simulink library "inp"  (R2021b)
settings: Solver=VariableStepAuto  StartTime=0.0  StopTime=10.0  RelTol=1e-3
undefined symbols (not defined in the file): C_TASK_5MS_S, FALSE, KINP_AcoreReadyToSlp_flg_ovrdflg, KINP_AcoreReadyToSlp_flg_ovrdval, KINP_AllowMovThd_OTA_enum_ovrdflg, KINP_AllowMovThd_OTA_enum_ovrdval, KINP_APSAngleTarget_Deg_ovrdflg, KINP_APSAngleTarget_Deg_ovrdval, KINP_APSDecReq_mps2_ovrdflg, KINP_APSDecReq_mps2_ovrdval, KINP_APSDecReqA_flg_ovrdflg, KINP_APSDecReqA_flg_ovrdval, KINP_APSDFLL_cm_ovrdflg, KINP_APSDFLL_cm_ovrdval, KINP_APSDFLR_cm_ovrdflg, KINP_APSDFLR_cm_ovrdval, KINP_APSDRLL_cm_ovrdflg, KINP_APSDRLL_cm_ovrdval, KINP_APSDRLR_cm_ovrdflg, KINP_APSDRLR_cm_ovrdval, KINP_APSExitCondition_enum_ovrdflg, KINP_APSExitCondition_enum_ovrdval, KINP_APSHWVer_enum_ovrdflg, KINP_APSHWVer_enum_ovrdval, KINP_APSProgressPCT_pct_ovrdflg, KINP_APSProgressPCT_pct_ovrdval, KINP_APSPwrReq_enum_ovrdflg, KINP_APSPwrReq_enum_ovrdval, KINP_APSReq_enum_ovrdflg, KINP_APSReq_enum_ovrdval, KINP_APSRQDisplay_enum_ovrdflg, KINP_APSRQDisplay_enum_ovrdval, KINP_APSRqEPASCtrl_flg_ovrdflg, KINP_APSRqEPASCtrl_flg_ovrdval, KINP_APSShiftPosnReq_enum_ovrdval, KINP_APSShiftPosnReq_enum_ovrflg, KINP_APSSpeedCMD_kph_ovrdval, KINP_APSSpeedCMD_kph_ovrflg, KINP_APSStaSystem_enum_ovrdflg, KINP_APSStaSystem_enum_ovrdval, KINP_APSSWVer_enum_ovrdflg, KINP_APSSWVer_enum_ovrdval, KINP_APSVMCReqA_flg_ovrdval, KINP_APSVMCReqA_flg_ovrflg, KINP_APSVRqEPASCtrl_flg_ovrdflg, KINP_APSVRqEPASCtrl_flg_ovrdval, KINP_AuxBattVolmV_mV_ovrdflg, KINP_AuxBattVolmV_mV_ovrdval, KINP_CAASSta_enum_ovrdflg, KINP_CAASSta_enum_ovrdval, KINP_CAASVMCReqA_flg_ovrdval, KINP_CAASVMCReqA_flg_ovrflg, KINP_CAN1BusOff_flg_ovrdflg, KINP_CAN1BusOff_flg_ovrdval, KINP_CAN2BusOff_flg_ovrdflg, KINP_CAN2BusOff_flg_ovrdval, KINP_CAN3BusOff_flg_ovrdflg, KINP_CAN3BusOff_flg_ovrdval, KINP_CAN4BusOff_flg_ovrdflg, KINP_CAN4BusOff_flg_ovrdval ... (+152)
libraries: FVT_lib x1035, hcu_lib x1
(part 19 of 33)

== system inp/INP/CAN3/SignalCheck/BMS6 ==
  BHAL_outputs : Inport
  inp_CanValid_bus : Inport  Port=2
  BMS6CSErr : FVT_lib/inp/can_signal_template  SystemSampleTime=-1  VariantActivationTime=update diagram  Latency=0  AutoFrameSizeCalculation=off
      link override defval: Value=KINP_BMS6CSErr_flg_defval
      link override ovrdflg: Value=KINP_BMS6CSErr_flg_ovrdflg
      link override ovrdval: Value=KINP_BMS6CSErr_flg_ovrdval
  BMS6RCErr : FVT_lib/inp/can_signal_template  SystemSampleTime=-1  VariantActivationTime=update diagram  Latency=0  AutoFrameSizeCalculation=off
      link override defval: Value=KINP_BMS6RCErr_flg_defval
      link override ovrdflg: Value=KINP_BMS6RCErr_flg_ovrdflg
      link override ovrdval: Value=KINP_BMS6RCErr_flg_ovrdval
  BMSChckSum : FVT_lib/inp/can_signal_template  SystemSampleTime=-1  VariantActivationTime=update diagram  Latency=0  AutoFrameSizeCalculation=off
      link override defval: Value=KINP_BMSChckSum_enum_defval
      link override ovrdflg: Value=KINP_BMSChckSum_enum_ovrdflg
      link override ovrdval: Value=KINP_BMSChckSum_enum_ovrdval
  BMSREADY : FVT_lib/inp/can_signal_template  SystemSampleTime=-1  VariantActivationTime=update diagram  Latency=0  AutoFrameSizeCalculation=off
      link override defval: Value=KINP_BMSREADY_flg_defval
      link override ovrdflg: Value=KINP_BMSREADY_flg_ovrdflg
      link override ovrdval: Value=KINP_BMSREADY_flg_ovrdval
  BMSRolCnct : FVT_lib/inp/can_signal_template  SystemSampleTime=-1  VariantActivationTime=update diagram  Latency=0  AutoFrameSizeCalculation=off
      link override defval: Value=KINP_BMSRolCnct_enum_defval
      link override ovrdflg: Value=KINP_BMSRolCnct_enum_ovrdflg
      link override ovrdval: Value=KINP_BMSRolCnct_enum_ovrdval
  BMSWarn1 : FVT_lib/inp/can_signal_template  SystemSampleTime=-1  VariantActivationTime=update diagram  Latency=0  AutoFrameSizeCalculation=off
      link override defval: Value=KINP_BMSWarn1_flg_defval
      link override ovrdflg: Value=KINP_BMSWarn1_flg_ovrdflg
      link override ovrdval: Value=KINP_BMSWarn1_flg_ovrdval
  BMSWarn2 : FVT_lib/inp/can_signal_template  SystemSampleTime=-1  VariantActivationTime=update diagram  Latency=0  AutoFrameSizeCalculation=off
      link override defval: Value=KINP_BMSWarn2_flg_defval
      link override ovrdflg: Value=KINP_BMSWarn2_flg_ovrdflg
      link override ovrdval: Value=KINP_BMSWarn2_flg_ovrdval
  BMSWarn3 : FVT_lib/inp/can_signal_template  SystemSampleTime=-1  VariantActivationTime=update diagram  Latency=0  AutoFrameSizeCalculation=off
      link override defval: Value=KINP_BMSWarn3_flg_defval
      link override ovrdflg: Value=KINP_BMSWarn3_flg_ovrdflg
      link override ovrdval: Value=KINP_BMSWarn3_flg_ovrdval
  BMSWarn4 : FVT_lib/inp/can_signal_template  SystemSampleTime=-1  VariantActivationTime=update diagram  Latency=0  AutoFrameSizeCalculation=off
      link override defval: Value=KINP_BMSWarn4_flg_defval
      link override ovrdflg: Value=KINP_BMSWarn4_flg_ovrdflg
      link override ovrdval: Value=KINP_BMSWarn4_flg_ovrdval
  BMSWarn5 : FVT_lib/inp/can_signal_template  SystemSampleTime=-1  VariantActivationTime=update diagram  Latency=0  AutoFrameSizeCalculation=off
      link override defval: Value=KINP_BMSWarn5_flg_defval
      link override ovrdflg: Value=KINP_BMSWarn5_flg_ovrdflg
      link override ovrdval: Value=KINP_BMSWarn5_flg_ovrdval
  BMSWarn6 : FVT_lib/inp/can_signal_template  SystemSampleTime=-1  VariantActivationTime=update diagram  Latency=0  AutoFrameSizeCalculation=off
      link override defval: Value=KINP_BMSWarn6_flg_defval
      link override ovrdflg: Value=KINP_BMSWarn6_flg_ovrdflg
      link override ovrdval: Value=KINP_BMSWarn6_flg_ovrdval
  BMSWarn7 : FVT_lib/inp/can_signal_template  SystemSampleTime=-1  VariantActivationTime=update diagram  Latency=0  AutoFrameSizeCalculation=off
      link override defval: Value=KINP_BMSWarn7_flg_defval
      link override ovrdflg: Value=KINP_BMSWarn7_flg_ovrdflg
      link override ovrdval: Value=KINP_BMSWarn7_flg_ovrdval
  BMSWarn8 : FVT_lib/inp/can_signal_template  SystemSampleTime=-1  VariantActivationTime=update diagram  Latency=0  AutoFrameSizeCalculation=off
      link override defval: Value=KINP_BMSWarn8_flg_defval
      link override ovrdflg: Value=KINP_BMSWarn8_flg_ovrdflg
      link override ovrdval: Value=KINP_BMSWarn8_flg_ovrdval
  ChrgInLockReq : FVT_lib/inp/can_signal_template  SystemSampleTime=-1  VariantActivationTime=update diagram  Latency=0  AutoFrameSizeCalculation=off
      link override defval: Value=KINP_ChrgInLockReq_enum_defval
      link override ovrdflg: Value=KINP_ChrgInLockReq_enum_ovrdflg
      link override ovrdval: Value=KINP_ChrgInLockReq_enum_ovrdval
  ChrgPlugSta : FVT_lib/inp/can_signal_template  SystemSampleTime=-1  VariantActivationTime=update diagram  Latency=0  AutoFrameSizeCalculation=off
      link override defval: Value=KINP_ChrgPlugSta_enum_defval
      link override ovrdflg: Value=KINP_ChrgPlugSta_enum_ovrdflg
      link override ovrdval: Value=KINP_ChrgPlugSta_enum_ovrdval
  DisChrgPlugErr : FVT_lib/inp/can_signal_template  SystemSampleTime=-1  VariantActivationTime=update diagram  Latency=0  AutoFrameSizeCalculation=off
      link override defval: Value=KINP_DisChrgPlugErr_enum_defval
      link override ovrdflg: Value=KINP_DisChrgPlugErr_enum_ovrdflg
      link override ovrdval: Value=KINP_DisChrgPlugErr_enum_ovrdval
  ExtChrgSta : FVT_lib/inp/can_signal_template  SystemSampleTime=-1  VariantActivationTime=update diagram  Latency=0  AutoFrameSizeCalculation=off
      link override defval: Value=KINP_ExtChrgSta_enum_defval
      link override ovrdflg: Value=KINP_ExtChrgSta_enum_ovrdflg
      link override ovrdval: Value=KINP_ExtChrgSta_enum_ovrdval
  HVBChrgErr : FVT_lib/inp/can_signal_template  SystemSampleTime=-1  VariantActivationTime=update diagram  Latency=0  AutoFrameSizeCalculation=off
      link override defval: Value=KINP_HVBChrgErr_enum_defval
      link override ovrdflg: Value=KINP_HVBChrgErr_enum_ovrdflg
      link override ovrdval: Value=KINP_HVBChrgErr_enum_ovrdval
  HVBContactorSta : FVT_lib/inp/can_signal_template  SystemSampleTime=-1  VariantActivationTime=update diagram  Latency=0  AutoFrameSizeCalculation=off
      link override defval: Value=KINP_HVBContactorSta_flg_defval
      link override ovrdflg: Value=KINP_HVBContactorSta_flg_ovrdflg
      link override ovrdval: Value=KINP_HVBContactorSta_flg_ovrdval
  HVBHVILErr : FVT_lib/inp/can_signal_template  SystemSampleTime=-1  VariantActivationTime=update diagram  Latency=0  AutoFrameSizeCalculation=off
      link override defval: Value=KINP_HVBHVILErr_flg_defval
      link override ovrdflg: Value=KINP_HVBHVILErr_flg_ovrdflg
      link override ovrdval: Value=KINP_HVBHVILErr_flg_ovrdval
  HVBOvrTempErr : FVT_lib/inp/can_signal_template  SystemSampleTime=-1  VariantActivationTime=update diagram  Latency=0  AutoFrameSizeCalculation=off
      link override defval: Value=KINP_HVBOvrTempErr_flg_defval
      link override ovrdflg: Value=KINP_HVBOvrTempErr_flg_ovrdflg
      link override ovrdval: Value=KINP_HVBOvrTempErr_flg_ovrdval
  HVBOvrTempWarn : FVT_lib/inp/can_signal_template  SystemSampleTime=-1  VariantActivationTime=update diagram  Latency=0  AutoFrameSizeCalculation=off
      link override defval: Value=KINP_HVBOvrTempWarn_enum_defval
      link override ovrdflg: Value=KINP_HVBOvrTempWarn_enum_ovrdflg
      link override ovrdval: Value=KINP_HVBOvrTempWarn_enum_ovrdval
  HVBPreheatPrecoolSta : FVT_lib/inp/can_signal_template  SystemSampleTime=-1  VariantActivationTime=update diagram  Latency=0  AutoFrameSizeCalculation=off
      link override defval: Value=KINP_HVBPreheatPrecoolSta_enum_defval
      link override ovrdflg: Value=KINP_HVBPreheatPrecoolSta_enum_ovrdflg
      link override ovrdval: Value=KINP_HVBPreheatPrecoolSta_enum_ovrdval
  HVBattReady4Pre : FVT_lib/inp/can_signal_template  SystemSampleTime=-1  VariantActivationTime=update diagram  Latency=0  AutoFrameSizeCalculation=off
      link override defval: Value=KINP_HVBattReady4Pre_enum_defval
      link override ovrdflg: Value=KINP_HVBattReady4Pre_enum_ovrdflg
      link override ovrdval: Value=KINP_HVBattReady4Pre_enum_ovrdval
  HVILSta : FVT_lib/inp/can_signal_template  SystemSampleTime=-1  VariantActivationTime=update diagram  Latency=0  AutoFrameSizeCalculation=off
      link override defval: Value=KINP_HVILSta_flg_defval
      link override ovrdflg: Value=KINP_HVILSta_flg_ovrdflg
      link override ovrdval: Value=KINP_HVILSta_flg_ovrdval
  Terminator_{1..26} (26 alike) : Terminator
  True_VHAL_BMS6CSErr_flg : Constant  Value=TRUE  OutDataTypeStr=boolean
  True_VHAL_BMS6RCErr_flg : Constant  Value=TRUE  OutDataTypeStr=boolean
  True_VHAL_BMSChckSum_enum : Constant  Value=TRUE  OutDataTypeStr=boolean
  True_VHAL_BMSREADY_flg : Constant  Value=TRUE  OutDataTypeStr=boolean
  True_VHAL_BMSRolCnct_enum : Constant  Value=TRUE  OutDataTypeStr=boolean
  True_VHAL_BMSWarn1_flg : Constant  Value=TRUE  OutDataTypeStr=boolean
  True_VHAL_BMSWarn2_flg : Constant  Value=TRUE  OutDataTypeStr=boolean
  True_VHAL_BMSWarn3_flg : Constant  Value=TRUE  OutDataTypeStr=boolean
  True_VHAL_BMSWarn4_flg : Constant  Value=TRUE  OutDataTypeStr=boolean
  True_VHAL_BMSWarn5_flg : Constant  Value=TRUE  OutDataTypeStr=boolean
  True_VHAL_BMSWarn6_flg : Constant  Value=TRUE  OutDataTypeStr=boolean
  True_VHAL_BMSWarn7_flg : Constant  Value=TRUE  OutDataTypeStr=boolean
  True_VHAL_BMSWarn8_flg : Constant  Value=TRUE  OutDataTypeStr=boolean
  True_VHAL_ChrgInLockReq_enum : Constant  Value=TRUE  OutDataTypeStr=boolean
  True_VHAL_ChrgPlugSta_enum : Constant  Value=TRUE  OutDataTypeStr=boolean
  True_VHAL_DisChrgPlugErr_enum : Constant  Value=TRUE  OutDataTypeStr=boolean
  True_VHAL_ExtChrgSta_enum : Constant  Value=TRUE  OutDataTypeStr=boolean
  True_VHAL_HVBChrgErr_enum : Constant  Value=TRUE  OutDataTypeStr=boolean
  True_VHAL_HVBContactorSta_flg : Constant  Value=TRUE  OutDataTypeStr=boolean
  True_VHAL_HVBHVILErr_flg : Constant  Value=TRUE  OutDataTypeStr=boolean
  True_VHAL_HVBOvrTempErr_flg : Constant  Value=TRUE  OutDataTypeStr=boolean
  True_VHAL_HVBOvrTempWarn_enum : Constant  Value=TRUE  OutDataTypeStr=boolean
  True_VHAL_HVBPreheatPrecoolSta_enum : Constant  Value=TRUE  OutDataTypeStr=boolean
  True_VHAL_HVBattReady4Pre_enum : Constant  Value=TRUE  OutDataTypeStr=boolean
  True_VHAL_HVILSta_flg : Constant  Value=TRUE  OutDataTypeStr=boolean
  True_VHAL_V2LSta_enum : Constant  Value=TRUE  OutDataTypeStr=boolean
  V2LSta : FVT_lib/inp/can_signal_template  SystemSampleTime=-1  VariantActivationTime=update diagram  Latency=0  AutoFrameSizeCalculation=off
      link override defval: Value=KINP_V2LSta_enum_defval
      link override ovrdflg: Value=KINP_V2LSta_enum_ovrdflg
      link override ovrdval: Value=KINP_V2LSta_enum_ovrdval
  slr1_{1..26} (26 alike) : BusSelector  OutputSignals=VINP_CANMsgValidBMS6_flg
  slr_VHAL_BMS6CSErr_flg : BusSelector  OutputSignals=VHAL_BMS6CSErr_flg
  slr_VHAL_BMS6RCErr_flg : BusSelector  OutputSignals=VHAL_BMS6RCErr_flg
  slr_VHAL_BMSChckSum_enum : BusSelector  OutputSignals=VHAL_BMSChckSum_enum
  slr_VHAL_BMSREADY_flg : BusSelector  OutputSignals=VHAL_BMSREADY_flg
  slr_VHAL_BMSRolCnct_enum : BusSelector  OutputSignals=VHAL_BMSRolCnct_enum
  slr_VHAL_BMSWarn1_flg : BusSelector  OutputSignals=VHAL_BMSWarn1_flg
  slr_VHAL_BMSWarn2_flg : BusSelector  OutputSignals=VHAL_BMSWarn2_flg
  slr_VHAL_BMSWarn3_flg : BusSelector  OutputSignals=VHAL_BMSWarn3_flg
  slr_VHAL_BMSWarn4_flg : BusSelector  OutputSignals=VHAL_BMSWarn4_flg
  slr_VHAL_BMSWarn5_flg : BusSelector  OutputSignals=VHAL_BMSWarn5_flg
  slr_VHAL_BMSWarn6_flg : BusSelector  OutputSignals=VHAL_BMSWarn6_flg
  slr_VHAL_BMSWarn7_flg : BusSelector  OutputSignals=VHAL_BMSWarn7_flg
  slr_VHAL_BMSWarn8_flg : BusSelector  OutputSignals=VHAL_BMSWarn8_flg
  slr_VHAL_ChrgInLockReq_enum : BusSelector  OutputSignals=VHAL_ChrgInLockReq_enum
  slr_VHAL_ChrgPlugSta_enum : BusSelector  OutputSignals=VHAL_ChrgPlugSta_enum
  slr_VHAL_DisChrgPlugErr_enum : BusSelector  OutputSignals=VHAL_DisChrgPlugErr_enum
  slr_VHAL_ExtChrgSta_enum : BusSelector  OutputSignals=VHAL_ExtChrgSta_enum
  slr_VHAL_HVBChrgErr_enum : BusSelector  OutputSignals=VHAL_HVBChrgErr_enum
  slr_VHAL_HVBContactorSta_flg : BusSelector  OutputSignals=VHAL_HVBContactorSta_flg
  slr_VHAL_HVBHVILErr_flg : BusSelector  OutputSignals=VHAL_HVBHVILErr_flg
  slr_VHAL_HVBOvrTempErr_flg : BusSelector  OutputSignals=VHAL_HVBOvrTempErr_flg
  slr_VHAL_HVBOvrTempWarn_enum : BusSelector  OutputSignals=VHAL_HVBOvrTempWarn_enum
  slr_VHAL_HVBPreheatPrecoolSta_enum : BusSelector  OutputSignals=VHAL_HVBPreheatPrecoolSta_enum
  slr_VHAL_HVBattReady4Pre_enum : BusSelector  OutputSignals=VHAL_HVBattReady4Pre_enum
  slr_VHAL_HVILSta_flg : BusSelector  OutputSignals=VHAL_HVILSta_flg
  slr_VHAL_V2LSta_enum : BusSelector  OutputSignals=VHAL_V2LSta_enum
  VINP_BMS6CSErr_flg : Outport
  VINP_BMS6RCErr_flg : Outport  Port=2
  VINP_BMSChckSum_enum : Outport  Port=3
  VINP_BMSRolCnct_enum : Outport  Port=4
  VINP_BMSREADY_flg : Outport  Port=5
  VINP_BMSWarn1_flg : Outport  Port=6
  VINP_BMSWarn2_flg : Outport  Port=7
  VINP_BMSWarn3_flg : Outport  Port=8
  VINP_BMSWarn4_flg : Outport  Port=9
  VINP_BMSWarn5_flg : Outport  Port=10
  VINP_BMSWarn6_flg : Outport  Port=11
  VINP_BMSWarn7_flg : Outport  Port=12
  VINP_BMSWarn8_flg : Outport  Port=13
  VINP_ChrgInLockReq_enum : Outport  Port=14
  VINP_ChrgPlugSta_enum : Outport  Port=15
  VINP_DisChrgPlugErr_enum : Outport  Port=16
  VINP_ExtChrgSta_enum : Outport  Port=17
  VINP_HVBChrgErr_enum : Outport  Port=18
  VINP_HVBContactorSta_flg : Outport  Port=19
  VINP_HVBHVILErr_flg : Outport  Port=20
  VINP_HVBOvrTempErr_flg : Outport  Port=21
  VINP_HVBOvrTempWarn_enum : Outport  Port=22
  VINP_HVBPreheatPrecoolSta_enum : Outport  Port=23
  VINP_HVBattReady4Pre_enum : Outport  Port=24
  VINP_HVILSta_flg : Outport  Port=25
  VINP_V2LSta_enum : Outport  Port=26
  wires:
  BHAL_outputs/1 -> [BHAL_outputs]
  inp_CanValid_bus/1 -> [inp_CanValid_bus]
  [BHAL_outputs] -> slr_VHAL_BMS6CSErr_flg/1
  slr_VHAL_BMS6CSErr_flg/1 -> BMS6CSErr/1  "<VHAL_BMS6CSErr_flg>"
  True_VHAL_BMS6CSErr_flg/1 -> BMS6CSErr/2
  [inp_CanValid_bus] -> slr1_1/1
  slr1_1/1 -> BMS6CSErr/3  "<VINP_CANMsgValidBMS6_flg>"
  BMS6CSErr/1 -> VINP_BMS6CSErr_flg/1  "VINP_BMS6CSErr_flg"
  BMS6CSErr/2 -> Terminator_1/1
  [BHAL_outputs] -> slr_VHAL_BMS6RCErr_flg/1
  slr_VHAL_BMS6RCErr_flg/1 -> BMS6RCErr/1  "<VHAL_BMS6RCErr_flg>"
  True_VHAL_BMS6RCErr_flg/1 -> BMS6RCErr/2
  [inp_CanValid_bus] -> slr1_2/1
  slr1_2/1 -> BMS6RCErr/3  "<VINP_CANMsgValidBMS6_flg>"
  BMS6RCErr/1 -> VINP_BMS6RCErr_flg/1  "VINP_BMS6RCErr_flg"
  BMS6RCErr/2 -> Terminator_2/1
  [BHAL_outputs] -> slr_VHAL_BMSChckSum_enum/1
  slr_VHAL_BMSChckSum_enum/1 -> BMSChckSum/1  "<VHAL_BMSChckSum_enum>"
  True_VHAL_BMSChckSum_enum/1 -> BMSChckSum/2
  [inp_CanValid_bus] -> slr1_3/1
  slr1_3/1 -> BMSChckSum/3  "<VINP_CANMsgValidBMS6_flg>"
  BMSChckSum/1 -> VINP_BMSChckSum_enum/1  "VINP_BMSChckSum_enum"
  BMSChckSum/2 -> Terminator_3/1
  [BHAL_outputs] -> slr_VHAL_BMSRolCnct_enum/1
  slr_VHAL_BMSRolCnct_enum/1 -> BMSRolCnct/1  "<VHAL_BMSRolCnct_enum>"
  True_VHAL_BMSRolCnct_enum/1 -> BMSRolCnct/2
  [inp_CanValid_bus] -> slr1_4/1
  slr1_4/1 -> BMSRolCnct/3  "<VINP_CANMsgValidBMS6_flg>"
  BMSRolCnct/1 -> VINP_BMSRolCnct_enum/1  "VINP_BMSRolCnct_enum"
  BMSRolCnct/2 -> Terminator_4/1
  [BHAL_outputs] -> slr_VHAL_BMSREADY_flg/1
  slr_VHAL_BMSREADY_flg/1 -> BMSREADY/1  "<VHAL_BMSREADY_flg>"
  True_VHAL_BMSREADY_flg/1 -> BMSREADY/2
  [inp_CanValid_bus] -> slr1_5/1
  slr1_5/1 -> BMSREADY/3  "<VINP_CANMsgValidBMS6_flg>"
  BMSREADY/1 -> VINP_BMSREADY_flg/1  "VINP_BMSREADY_flg"
  BMSREADY/2 -> Terminator_5/1
  [BHAL_outputs] -> slr_VHAL_BMSWarn1_flg/1
  slr_VHAL_BMSWarn1_flg/1 -> BMSWarn1/1  "<VHAL_BMSWarn1_flg>"
  True_VHAL_BMSWarn1_flg/1 -> BMSWarn1/2
  [inp_CanValid_bus] -> slr1_6/1
  slr1_6/1 -> BMSWarn1/3  "<VINP_CANMsgValidBMS6_flg>"
  BMSWarn1/1 -> VINP_BMSWarn1_flg/1  "VINP_BMSWarn1_flg"
  BMSWarn1/2 -> Terminator_6/1
  [BHAL_outputs] -> slr_VHAL_BMSWarn2_flg/1
  slr_VHAL_BMSWarn2_flg/1 -> BMSWarn2/1  "<VHAL_BMSWarn2_flg>"
  True_VHAL_BMSWarn2_flg/1 -> BMSWarn2/2
  [inp_CanValid_bus] -> slr1_7/1
  slr1_7/1 -> BMSWarn2/3  "<VINP_CANMsgValidBMS6_flg>"
  BMSWarn2/1 -> VINP_BMSWarn2_flg/1  "VINP_BMSWarn2_flg"
  BMSWarn2/2 -> Terminator_7/1
  [BHAL_outputs] -> slr_VHAL_BMSWarn3_flg/1
  slr_VHAL_BMSWarn3_flg/1 -> BMSWarn3/1  "<VHAL_BMSWarn3_flg>"
  True_VHAL_BMSWarn3_flg/1 -> BMSWarn3/2
  [inp_CanValid_bus] -> slr1_8/1
  slr1_8/1 -> BMSWarn3/3  "<VINP_CANMsgValidBMS6_flg>"
  BMSWarn3/1 -> VINP_BMSWarn3_flg/1  "VINP_BMSWarn3_flg"
  BMSWarn3/2 -> Terminator_8/1
  [BHAL_outputs] -> slr_VHAL_BMSWarn4_flg/1
  slr_VHAL_BMSWarn4_flg/1 -> BMSWarn4/1  "<VHAL_BMSWarn4_flg>"
  True_VHAL_BMSWarn4_flg/1 -> BMSWarn4/2
  [inp_CanValid_bus] -> slr1_9/1
  slr1_9/1 -> BMSWarn4/3  "<VINP_CANMsgValidBMS6_flg>"
  BMSWarn4/1 -> VINP_BMSWarn4_flg/1  "VINP_BMSWarn4_flg"
  BMSWarn4/2 -> Terminator_9/1
  [BHAL_outputs] -> slr_VHAL_BMSWarn5_flg/1
  slr_VHAL_BMSWarn5_flg/1 -> BMSWarn5/1  "<VHAL_BMSWarn5_flg>"
  True_VHAL_BMSWarn5_flg/1 -> BMSWarn5/2
  [inp_CanValid_bus] -> slr1_10/1
  slr1_10/1 -> BMSWarn5/3  "<VINP_CANMsgValidBMS6_flg>"
  BMSWarn5/1 -> VINP_BMSWarn5_flg/1  "VINP_BMSWarn5_flg"
  BMSWarn5/2 -> Terminator_10/1
  [BHAL_outputs] -> slr_VHAL_BMSWarn6_flg/1
  slr_VHAL_BMSWarn6_flg/1 -> BMSWarn6/1  "<VHAL_BMSWarn6_flg>"
  True_VHAL_BMSWarn6_flg/1 -> BMSWarn6/2
  [inp_CanValid_bus] -> slr1_11/1
  slr1_11/1 -> BMSWarn6/3  "<VINP_CANMsgValidBMS6_flg>"
  BMSWarn6/1 -> VINP_BMSWarn6_flg/1  "VINP_BMSWarn6_flg"
  BMSWarn6/2 -> Terminator_11/1
  [BHAL_outputs] -> slr_VHAL_BMSWarn7_flg/1
  slr_VHAL_BMSWarn7_flg/1 -> BMSWarn7/1  "<VHAL_BMSWarn7_flg>"
  True_VHAL_BMSWarn7_flg/1 -> BMSWarn7/2
  [inp_CanValid_bus] -> slr1_12/1
  slr1_12/1 -> BMSWarn7/3  "<VINP_CANMsgValidBMS6_flg>"
  BMSWarn7/1 -> VINP_BMSWarn7_flg/1  "VINP_BMSWarn7_flg"
  BMSWarn7/2 -> Terminator_12/1
  [BHAL_outputs] -> slr_VHAL_BMSWarn8_flg/1
  slr_VHAL_BMSWarn8_flg/1 -> BMSWarn8/1  "<VHAL_BMSWarn8_flg>"
  True_VHAL_BMSWarn8_flg/1 -> BMSWarn8/2
  [inp_CanValid_bus] -> slr1_13/1
  slr1_13/1 -> BMSWarn8/3  "<VINP_CANMsgValidBMS6_flg>"
  BMSWarn8/1 -> VINP_BMSWarn8_flg/1  "VINP_BMSWarn8_flg"
  BMSWarn8/2 -> Terminator_13/1
  [BHAL_outputs] -> slr_VHAL_ChrgInLockReq_enum/1
  slr_VHAL_ChrgInLockReq_enum/1 -> ChrgInLockReq/1  "<VHAL_ChrgInLockReq_enum>"
  True_VHAL_ChrgInLockReq_enum/1 -> ChrgInLockReq/2
  [inp_CanValid_bus] -> slr1_14/1
  slr1_14/1 -> ChrgInLockReq/3  "<VINP_CANMsgValidBMS6_flg>"
  ChrgInLockReq/1 -> VINP_ChrgInLockReq_enum/1  "VINP_ChrgInLockReq_enum"
  ChrgInLockReq/2 -> Terminator_14/1
  [BHAL_outputs] -> slr_VHAL_ChrgPlugSta_enum/1
  slr_VHAL_ChrgPlugSta_enum/1 -> ChrgPlugSta/1  "<VHAL_ChrgPlugSta_enum>"
  True_VHAL_ChrgPlugSta_enum/1 -> ChrgPlugSta/2
  [inp_CanValid_bus] -> slr1_15/1
  slr1_15/1 -> ChrgPlugSta/3  "<VINP_CANMsgValidBMS6_flg>"
  ChrgPlugSta/1 -> VINP_ChrgPlugSta_enum/1  "VINP_ChrgPlugSta_enum"
  ChrgPlugSta/2 -> Terminator_15/1
  [BHAL_outputs] -> slr_VHAL_DisChrgPlugErr_enum/1
  slr_VHAL_DisChrgPlugErr_enum/1 -> DisChrgPlugErr/1  "<VHAL_DisChrgPlugErr_enum>"
  True_VHAL_DisChrgPlugErr_enum/1 -> DisChrgPlugErr/2
  [inp_CanValid_bus] -> slr1_16/1
  slr1_16/1 -> DisChrgPlugErr/3  "<VINP_CANMsgValidBMS6_flg>"
  DisChrgPlugErr/1 -> VINP_DisChrgPlugErr_enum/1  "VINP_DisChrgPlugErr_enum"
  DisChrgPlugErr/2 -> Terminator_16/1
  [BHAL_outputs] -> slr_VHAL_ExtChrgSta_enum/1
  slr_VHAL_ExtChrgSta_enum/1 -> ExtChrgSta/1  "<VHAL_ExtChrgSta_enum>"
  True_VHAL_ExtChrgSta_enum/1 -> ExtChrgSta/2
  [inp_CanValid_bus] -> slr1_17/1
  slr1_17/1 -> ExtChrgSta/3  "<VINP_CANMsgValidBMS6_flg>"
  ExtChrgSta/1 -> VINP_ExtChrgSta_enum/1  "VINP_ExtChrgSta_enum"
  ExtChrgSta/2 -> Terminator_17/1
  [BHAL_outputs] -> slr_VHAL_HVBChrgErr_enum/1
  slr_VHAL_HVBChrgErr_enum/1 -> HVBChrgErr/1  "<VHAL_HVBChrgErr_enum>"
  True_VHAL_HVBChrgErr_enum/1 -> HVBChrgErr/2
  [inp_CanValid_bus] -> slr1_18/1
  slr1_18/1 -> HVBChrgErr/3  "<VINP_CANMsgValidBMS6_flg>"
  HVBChrgErr/1 -> VINP_HVBChrgErr_enum/1  "VINP_HVBChrgErr_enum"
  HVBChrgErr/2 -> Terminator_18/1
  [BHAL_outputs] -> slr_VHAL_HVBContactorSta_flg/1
  slr_VHAL_HVBContactorSta_flg/1 -> HVBContactorSta/1  "<VHAL_HVBContactorSta_flg>"
  True_VHAL_HVBContactorSta_flg/1 -> HVBContactorSta/2
  [inp_CanValid_bus] -> slr1_19/1
  slr1_19/1 -> HVBContactorSta/3  "<VINP_CANMsgValidBMS6_flg>"
  HVBContactorSta/1 -> VINP_HVBContactorSta_flg/1  "VINP_HVBContactorSta_flg"
  HVBContactorSta/2 -> Terminator_19/1
  [BHAL_outputs] -> slr_VHAL_HVBHVILErr_flg/1
  slr_VHAL_HVBHVILErr_flg/1 -> HVBHVILErr/1  "<VHAL_HVBHVILErr_flg>"
  True_VHAL_HVBHVILErr_flg/1 -> HVBHVILErr/2
  [inp_CanValid_bus] -> slr1_20/1
  slr1_20/1 -> HVBHVILErr/3  "<VINP_CANMsgValidBMS6_flg>"
  HVBHVILErr/1 -> VINP_HVBHVILErr_flg/1  "VINP_HVBHVILErr_flg"
  HVBHVILErr/2 -> Terminator_20/1
  [BHAL_outputs] -> slr_VHAL_HVBOvrTempErr_flg/1
  slr_VHAL_HVBOvrTempErr_flg/1 -> HVBOvrTempErr/1  "<VHAL_HVBOvrTempErr_flg>"
  True_VHAL_HVBOvrTempErr_flg/1 -> HVBOvrTempErr/2
  [inp_CanValid_bus] -> slr1_21/1
  slr1_21/1 -> HVBOvrTempErr/3  "<VINP_CANMsgValidBMS6_flg>"
  HVBOvrTempErr/1 -> VINP_HVBOvrTempErr_flg/1  "VINP_HVBOvrTempErr_flg"
  HVBOvrTempErr/2 -> Terminator_21/1
  [BHAL_outputs] -> slr_VHAL_HVBOvrTempWarn_enum/1
  slr_VHAL_HVBOvrTempWarn_enum/1 -> HVBOvrTempWarn/1  "<VHAL_HVBOvrTempWarn_enum>"
  True_VHAL_HVBOvrTempWarn_enum/1 -> HVBOvrTempWarn/2
  [inp_CanValid_bus] -> slr1_22/1
  slr1_22/1 -> HVBOvrTempWarn/3  "<VINP_CANMsgValidBMS6_flg>"
  HVBOvrTempWarn/1 -> VINP_HVBOvrTempWarn_enum/1  "VINP_HVBOvrTempWarn_enum"
  HVBOvrTempWarn/2 -> Terminator_22/1
  [BHAL_outputs] -> slr_VHAL_HVBPreheatPrecoolSta_enum/1
  slr_VHAL_HVBPreheatPrecoolSta_enum/1 -> HVBPreheatPrecoolSta/1  "<VHAL_HVBPreheatPrecoolSta_enum>"
  True_VHAL_HVBPreheatPrecoolSta_enum/1 -> HVBPreheatPrecoolSta/2
  [inp_CanValid_bus] -> slr1_23/1
  slr1_23/1 -> HVBPreheatPrecoolSta/3  "<VINP_CANMsgValidBMS6_flg>"
  HVBPreheatPrecoolSta/1 -> VINP_HVBPreheatPrecoolSta_enum/1  "VINP_HVBPreheatPrecoolSta_enum"
  HVBPreheatPrecoolSta/2 -> Terminator_23/1
  [BHAL_outputs] -> slr_VHAL_HVBattReady4Pre_enum/1
  slr_VHAL_HVBattReady4Pre_enum/1 -> HVBattReady4Pre/1  "<VHAL_HVBattReady4Pre_enum>"
  True_VHAL_HVBattReady4Pre_enum/1 -> HVBattReady4Pre/2
  [inp_CanValid_bus] -> slr1_24/1
  slr1_24/1 -> HVBattReady4Pre/3  "<VINP_CANMsgValidBMS6_flg>"
  HVBattReady4Pre/1 -> VINP_HVBattReady4Pre_enum/1  "VINP_HVBattReady4Pre_enum"
  HVBattReady4Pre/2 -> Terminator_24/1
  [BHAL_outputs] -> slr_VHAL_HVILSta_flg/1
  slr_VHAL_HVILSta_flg/1 -> HVILSta/1  "<VHAL_HVILSta_flg>"
  True_VHAL_HVILSta_flg/1 -> HVILSta/2
  [inp_CanValid_bus] -> slr1_25/1
  slr1_25/1 -> HVILSta/3  "<VINP_CANMsgValidBMS6_flg>"
  HVILSta/1 -> VINP_HVILSta_flg/1  "VINP_HVILSta_flg"
  HVILSta/2 -> Terminator_25/1
  [BHAL_outputs] -> slr_VHAL_V2LSta_enum/1
  slr_VHAL_V2LSta_enum/1 -> V2LSta/1  "<VHAL_V2LSta_enum>"
  True_VHAL_V2LSta_enum/1 -> V2LSta/2
  [inp_CanValid_bus] -> slr1_26/1
  slr1_26/1 -> V2LSta/3  "<VINP_CANMsgValidBMS6_flg>"
  V2LSta/1 -> VINP_V2LSta_enum/1  "VINP_V2LSta_enum"
  V2LSta/2 -> Terminator_26/1

== system inp/INP/CAN3/SignalCheck/BMS8 ==
  BHAL_outputs : Inport
  inp_CanValid_bus : Inport  Port=2
  MainRlyNegSta : FVT_lib/inp/can_signal_template  SystemSampleTime=-1  VariantActivationTime=update diagram  Latency=0  AutoFrameSizeCalculation=off
      link override defval: Value=KINP_MainRlyNegSta_enum_defval
      link override ovrdflg: Value=KINP_MainRlyNegSta_enum_ovrdflg
      link override ovrdval: Value=KINP_MainRlyNegSta_enum_ovrdval
  MainRlyPosSta : FVT_lib/inp/can_signal_template  SystemSampleTime=-1  VariantActivationTime=update diagram  Latency=0  AutoFrameSizeCalculation=off
      link override defval: Value=KINP_MainRlyPosSta_enum_defval
      link override ovrdflg: Value=KINP_MainRlyPosSta_enum_ovrdflg
      link override ovrdval: Value=KINP_MainRlyPosSta_enum_ovrdval
  Terminator_1 : Terminator
  Terminator_2 : Terminator
  True_VHAL_MainRlyNegSta_enum : Constant  Value=TRUE  OutDataTypeStr=boolean
  True_VHAL_MainRlyPosSta_enum : Constant  Value=TRUE  OutDataTypeStr=boolean
  slr1_1 : BusSelector  OutputSignals=VINP_CANMsgValidBMS8_flg
  slr1_2 : BusSelector  OutputSignals=VINP_CANMsgValidBMS8_flg
  slr_VHAL_MainRlyNegSta_enum : BusSelector  OutputSignals=VHAL_MainRlyNegSta_enum
  slr_VHAL_MainRlyPosSta_enum : BusSelector  OutputSignals=VHAL_MainRlyPosSta_enum
  VINP_MainRlyNegSta_enum : Outport
  VINP_MainRlyPosSta_enum : Outport  Port=2
  wires:
  BHAL_outputs/1 -> [BHAL_outputs]
  inp_CanValid_bus/1 -> [inp_CanValid_bus]
  [BHAL_outputs] -> slr_VHAL_MainRlyNegSta_enum/1
  slr_VHAL_MainRlyNegSta_enum/1 -> MainRlyNegSta/1  "<VHAL_MainRlyNegSta_enum>"
  True_VHAL_MainRlyNegSta_enum/1 -> MainRlyNegSta/2
  [inp_CanValid_bus] -> slr1_1/1
  slr1_1/1 -> MainRlyNegSta/3  "<VINP_CANMsgValidBMS8_flg>"
  MainRlyNegSta/1 -> VINP_MainRlyNegSta_enum/1  "VINP_MainRlyNegSta_enum"
  MainRlyNegSta/2 -> Terminator_1/1
  [BHAL_outputs] -> slr_VHAL_MainRlyPosSta_enum/1
  slr_VHAL_MainRlyPosSta_enum/1 -> MainRlyPosSta/1  "<VHAL_MainRlyPosSta_enum>"
  True_VHAL_MainRlyPosSta_enum/1 -> MainRlyPosSta/2
  [inp_CanValid_bus] -> slr1_2/1
  slr1_2/1 -> MainRlyPosSta/3  "<VINP_CANMsgValidBMS8_flg>"
  MainRlyPosSta/1 -> VINP_MainRlyPosSta_enum/1  "VINP_MainRlyPosSta_enum"
  MainRlyPosSta/2 -> Terminator_2/1

== system inp/INP/CAN3/SignalCheck/CCU1 ==
  BHAL_outputs : Inport
  inp_CanValid_bus : Inport  Port=2
  CCU1CSErr : FVT_lib/inp/can_signal_template  SystemSampleTime=-1  VariantActivationTime=update diagram  Latency=0  AutoFrameSizeCalculation=off
      link override defval: Value=KINP_CCU1CSErr_flg_defval
      link override ovrdflg: Value=KINP_CCU1CSErr_flg_ovrdflg
      link override ovrdval: Value=KINP_CCU1CSErr_flg_ovrdval
  CCU1RCErr : FVT_lib/inp/can_signal_template  SystemSampleTime=-1  VariantActivationTime=update diagram  Latency=0  AutoFrameSizeCalculation=off
      link override defval: Value=KINP_CCU1RCErr_flg_defval
      link override ovrdflg: Value=KINP_CCU1RCErr_flg_ovrdflg
      link override ovrdval: Value=KINP_CCU1RCErr_flg_ovrdval
  CSCCU1 : FVT_lib/inp/can_signal_template  SystemSampleTime=-1  VariantActivationTime=update diagram  Latency=0  AutoFrameSizeCalculation=off
      link override defval: Value=KINP_CSCCU1_enum_defval
      link override ovrdflg: Value=KINP_CSCCU1_enum_ovrdflg
      link override ovrdval: Value=KINP_CSCCU1_enum_ovrdval
  DCDCAuxCur : FVT_lib/inp/can_signal_template  SystemSampleTime=-1  VariantActivationTime=update diagram  Latency=0  AutoFrameSizeCalculation=off
      link override defval: Value=KINP_DCDCAuxCur_A_defval
      link override ovrdflg: Value=KINP_DCDCAuxCur_A_ovrdflg
      link override ovrdval: Value=KINP_DCDCAuxCur_A_ovrdval
  DCDCAuxVolt : FVT_lib/inp/can_signal_template  SystemSampleTime=-1  VariantActivationTime=update diagram  Latency=0  AutoFrameSizeCalculation=off
      link override defval: Value=KINP_DCDCAuxVolt_V_defval
      link override ovrdflg: Value=KINP_DCDCAuxVolt_V_ovrdflg
      link override ovrdval: Value=KINP_DCDCAuxVolt_V_ovrdval
  DCDCHVCur : FVT_lib/inp/can_signal_template  SystemSampleTime=-1  VariantActivationTime=update diagram  Latency=0  AutoFrameSizeCalculation=off
      link override defval: Value=KINP_DCDCHVCur_A_defval
      link override ovrdflg: Value=KINP_DCDCHVCur_A_ovrdflg
      link override ovrdval: Value=KINP_DCDCHVCur_A_ovrdval
  DCDCInVoltInf : FVT_lib/inp/can_signal_template  SystemSampleTime=-1  VariantActivationTime=update diagram  Latency=0  AutoFrameSizeCalculation=off
      link override defval: Value=KINP_DCDCInVoltInf_V_defval
      link override ovrdflg: Value=KINP_DCDCInVoltInf_V_ovrdflg
      link override ovrdval: Value=KINP_DCDCInVoltInf_V_ovrdval
  DCDCPreCompleted : FVT_lib/inp/can_signal_template  SystemSampleTime=-1  VariantActivationTime=update diagram  Latency=0  AutoFrameSizeCalculation=off
      link override defval: Value=KINP_DCDCPreCompleted_enum_defval
      link override ovrdflg: Value=KINP_DCDCPreCompleted_enum_ovrdflg
      link override ovrdval: Value=KINP_DCDCPreCompleted_enum_ovrdval
  OBCDCCurrInf : FVT_lib/inp/can_signal_template  SystemSampleTime=-1  VariantActivationTime=update diagram  Latency=0  AutoFrameSizeCalculation=off
      link override defval: Value=KINP_OBCDCCurrInf_A_defval
      link override ovrdflg: Value=KINP_OBCDCCurrInf_A_ovrdflg
      link override ovrdval: Value=KINP_OBCDCCurrInf_A_ovrdval
  OBCDCVoltInf : FVT_lib/inp/can_signal_template  SystemSampleTime=-1  VariantActivationTime=update diagram  Latency=0  AutoFrameSizeCalculation=off
      link override defval: Value=KINP_OBCDCVoltInf_V_defval
      link override ovrdflg: Value=KINP_OBCDCVoltInf_V_ovrdflg
      link override ovrdval: Value=KINP_OBCDCVoltInf_V_ovrdval
  OBCPreCompleted : FVT_lib/inp/can_signal_template  SystemSampleTime=-1  VariantActivationTime=update diagram  Latency=0  AutoFrameSizeCalculation=off
      link override defval: Value=KINP_OBCPreCompleted_enum_defval
      link override ovrdflg: Value=KINP_OBCPreCompleted_enum_ovrdflg
      link override ovrdval: Value=KINP_OBCPreCompleted_enum_ovrdval
  OBCWakeup4Plugin : FVT_lib/inp/can_signal_template  SystemSampleTime=-1  VariantActivationTime=update diagram  Latency=0  AutoFrameSizeCalculation=off
      link override defval: Value=KINP_OBCWakeup4Plugin_flg_defval
      link override ovrdflg: Value=KINP_OBCWakeup4Plugin_flg_ovrdflg
      link override ovrdval: Value=KINP_OBCWakeup4Plugin_flg_ovrdval
  RCCCU1 : FVT_lib/inp/can_signal_template  SystemSampleTime=-1  VariantActivationTime=update diagram  Latency=0  AutoFrameSizeCalculation=off
      link override defval: Value=KINP_RCCCU1_enum_defval
      link override ovrdflg: Value=KINP_RCCCU1_enum_ovrdflg
      link override ovrdval: Value=KINP_RCCCU1_enum_ovrdval
  Terminator_{1..13} (13 alike) : Terminator
  True_VHAL_CCU1CSErr_flg : Constant  Value=TRUE  OutDataTypeStr=boolean
  True_VHAL_CCU1RCErr_flg : Constant  Value=TRUE  OutDataTypeStr=boolean
  True_VHAL_CSCCU1_enum : Constant  Value=TRUE  OutDataTypeStr=boolean
  True_VHAL_DCDCAuxCur_A : Constant  Value=TRUE  OutDataTypeStr=boolean
  True_VHAL_DCDCAuxVolt_V : Constant  Value=TRUE  OutDataTypeStr=boolean
  True_VHAL_DCDCHVCur_A : Constant  Value=TRUE  OutDataTypeStr=boolean
  True_VHAL_DCDCInVoltInf_V : Constant  Value=TRUE  OutDataTypeStr=boolean
  True_VHAL_DCDCPreCompleted_enum : Constant  Value=TRUE  OutDataTypeStr=boolean
  True_VHAL_OBCDCCurrInf_A : Constant  Value=TRUE  OutDataTypeStr=boolean
  True_VHAL_OBCDCVoltInf_V : Constant  Value=TRUE  OutDataTypeStr=boolean
  True_VHAL_OBCPreCompleted_enum : Constant  Value=TRUE  OutDataTypeStr=boolean
  True_VHAL_OBCWakeup4Plugin_flg : Constant  Value=TRUE  OutDataTypeStr=boolean
  True_VHAL_RCCCU1_enum : Constant  Value=TRUE  OutDataTypeStr=boolean
  slr1_{1..13} (13 alike) : BusSelector  OutputSignals=VINP_CANMsgValidCCU1_flg
  slr_VHAL_CCU1CSErr_flg : BusSelector  OutputSignals=VHAL_CCU1CSErr_flg
  slr_VHAL_CCU1RCErr_flg : BusSelector  OutputSignals=VHAL_CCU1RCErr_flg
  slr_VHAL_CSCCU1_enum : BusSelector  OutputSignals=VHAL_CSCCU1_enum
  slr_VHAL_DCDCAuxCur_A : BusSelector  OutputSignals=VHAL_DCDCAuxCur_A
  slr_VHAL_DCDCAuxVolt_V : BusSelector  OutputSignals=VHAL_DCDCAuxVolt_V
  slr_VHAL_DCDCHVCur_A : BusSelector  OutputSignals=VHAL_DCDCHVCur_A
  slr_VHAL_DCDCInVoltInf_V : BusSelector  OutputSignals=VHAL_DCDCInVoltInf_V
  slr_VHAL_DCDCPreCompleted_enum : BusSelector  OutputSignals=VHAL_DCDCPreCompleted_enum
  slr_VHAL_OBCDCCurrInf_A : BusSelector  OutputSignals=VHAL_OBCDCCurrInf_A
  slr_VHAL_OBCDCVoltInf_V : BusSelector  OutputSignals=VHAL_OBCDCVoltInf_V
  slr_VHAL_OBCPreCompleted_enum : BusSelector  OutputSignals=VHAL_OBCPreCompleted_enum
  slr_VHAL_OBCWakeup4Plugin_flg : BusSelector  OutputSignals=VHAL_OBCWakeup4Plugin_flg
  slr_VHAL_RCCCU1_enum : BusSelector  OutputSignals=VHAL_RCCCU1_enum
  VINP_CCU1CSErr_flg : Outport
  VINP_CCU1RCErr_flg : Outport  Port=2
  VINP_CSCCU1_enum : Outport  Port=3
  VINP_DCDCAuxCur_A : Outport  Port=4
  VINP_DCDCAuxVolt_V : Outport  Port=5
  VINP_DCDCHVCur_A : Outport  Port=6
  VINP_DCDCInVoltInf_V : Outport  Port=7
  VINP_DCDCPreCompleted_enum : Outport  Port=8
  VINP_OBCDCCurrInf_A : Outport  Port=9
  VINP_OBCDCVoltInf_V : Outport  Port=10
  VINP_OBCPreCompleted_enum : Outport  Port=11
  VINP_OBCWakeup4Plugin_flg : Outport  Port=12
  VINP_RCCCU1_enum : Outport  Port=13
  wires:
  BHAL_outputs/1 -> [BHAL_outputs]
  inp_CanValid_bus/1 -> [inp_CanValid_bus]
  [BHAL_outputs] -> slr_VHAL_CCU1CSErr_flg/1
  slr_VHAL_CCU1CSErr_flg/1 -> CCU1CSErr/1  "<VHAL_CCU1CSErr_flg>"
  True_VHAL_CCU1CSErr_flg/1 -> CCU1CSErr/2
  [inp_CanValid_bus] -> slr1_1/1
  slr1_1/1 -> CCU1CSErr/3  "<VINP_CANMsgValidCCU1_flg>"
  CCU1CSErr/1 -> VINP_CCU1CSErr_flg/1  "VINP_CCU1CSErr_flg"
  CCU1CSErr/2 -> Terminator_1/1
  [BHAL_outputs] -> slr_VHAL_CCU1RCErr_flg/1
  slr_VHAL_CCU1RCErr_flg/1 -> CCU1RCErr/1  "<VHAL_CCU1RCErr_flg>"
  True_VHAL_CCU1RCErr_flg/1 -> CCU1RCErr/2
  [inp_CanValid_bus] -> slr1_2/1
  slr1_2/1 -> CCU1RCErr/3  "<VINP_CANMsgValidCCU1_flg>"
  CCU1RCErr/1 -> VINP_CCU1RCErr_flg/1  "VINP_CCU1RCErr_flg"
  CCU1RCErr/2 -> Terminator_2/1
  [BHAL_outputs] -> slr_VHAL_CSCCU1_enum/1
  slr_VHAL_CSCCU1_enum/1 -> CSCCU1/1  "<VHAL_CSCCU1_enum>"
  True_VHAL_CSCCU1_enum/1 -> CSCCU1/2
  [inp_CanValid_bus] -> slr1_3/1
  slr1_3/1 -> CSCCU1/3  "<VINP_CANMsgValidCCU1_flg>"
  CSCCU1/1 -> VINP_CSCCU1_enum/1  "VINP_CSCCU1_enum"
  CSCCU1/2 -> Terminator_3/1
  [BHAL_outputs] -> slr_VHAL_DCDCAuxCur_A/1
  slr_VHAL_DCDCAuxCur_A/1 -> DCDCAuxCur/1  "<VHAL_DCDCAuxCur_A>"
  True_VHAL_DCDCAuxCur_A/1 -> DCDCAuxCur/2
  [inp_CanValid_bus] -> slr1_4/1
  slr1_4/1 -> DCDCAuxCur/3  "<VINP_CANMsgValidCCU1_flg>"
  DCDCAuxCur/1 -> VINP_DCDCAuxCur_A/1  "VINP_DCDCAuxCur_A"
  DCDCAuxCur/2 -> Terminator_4/1
  [BHAL_outputs] -> slr_VHAL_DCDCAuxVolt_V/1
  slr_VHAL_DCDCAuxVolt_V/1 -> DCDCAuxVolt/1  "<VHAL_DCDCAuxVolt_V>"
  True_VHAL_DCDCAuxVolt_V/1 -> DCDCAuxVolt/2
  [inp_CanValid_bus] -> slr1_5/1
  slr1_5/1 -> DCDCAuxVolt/3  "<VINP_CANMsgValidCCU1_flg>"
  DCDCAuxVolt/1 -> VINP_DCDCAuxVolt_V/1  "VINP_DCDCAuxVolt_V"
  DCDCAuxVolt/2 -> Terminator_5/1
  [BHAL_outputs] -> slr_VHAL_DCDCHVCur_A/1
  slr_VHAL_DCDCHVCur_A/1 -> DCDCHVCur/1  "<VHAL_DCDCHVCur_A>"
  True_VHAL_DCDCHVCur_A/1 -> DCDCHVCur/2
  [inp_CanValid_bus] -> slr1_6/1
  slr1_6/1 -> DCDCHVCur/3  "<VINP_CANMsgValidCCU1_flg>"
  DCDCHVCur/1 -> VINP_DCDCHVCur_A/1  "VINP_DCDCHVCur_A"
  DCDCHVCur/2 -> Terminator_6/1
  [BHAL_outputs] -> slr_VHAL_DCDCInVoltInf_V/1
  slr_VHAL_DCDCInVoltInf_V/1 -> DCDCInVoltInf/1  "<VHAL_DCDCInVoltInf_V>"
  True_VHAL_DCDCInVoltInf_V/1 -> DCDCInVoltInf/2
  [inp_CanValid_bus] -> slr1_7/1
  slr1_7/1 -> DCDCInVoltInf/3  "<VINP_CANMsgValidCCU1_flg>"
  DCDCInVoltInf/1 -> VINP_DCDCInVoltInf_V/1  "VINP_DCDCInVoltInf_V"
  DCDCInVoltInf/2 -> Terminator_7/1
  [BHAL_outputs] -> slr_VHAL_DCDCPreCompleted_enum/1
  slr_VHAL_DCDCPreCompleted_enum/1 -> DCDCPreCompleted/1  "<VHAL_DCDCPreCompleted_enum>"
  True_VHAL_DCDCPreCompleted_enum/1 -> DCDCPreCompleted/2
  [inp_CanValid_bus] -> slr1_8/1
  slr1_8/1 -> DCDCPreCompleted/3  "<VINP_CANMsgValidCCU1_flg>"
  DCDCPreCompleted/1 -> VINP_DCDCPreCompleted_enum/1  "VINP_DCDCPreCompleted_enum"
  DCDCPreCompleted/2 -> Terminator_8/1
  [BHAL_outputs] -> slr_VHAL_OBCDCCurrInf_A/1
  slr_VHAL_OBCDCCurrInf_A/1 -> OBCDCCurrInf/1  "<VHAL_OBCDCCurrInf_A>"
  True_VHAL_OBCDCCurrInf_A/1 -> OBCDCCurrInf/2
  [inp_CanValid_bus] -> slr1_9/1
  slr1_9/1 -> OBCDCCurrInf/3  "<VINP_CANMsgValidCCU1_flg>"
  OBCDCCurrInf/1 -> VINP_OBCDCCurrInf_A/1  "VINP_OBCDCCurrInf_A"
  OBCDCCurrInf/2 -> Terminator_9/1
  [BHAL_outputs] -> slr_VHAL_OBCDCVoltInf_V/1
  slr_VHAL_OBCDCVoltInf_V/1 -> OBCDCVoltInf/1  "<VHAL_OBCDCVoltInf_V>"
  True_VHAL_OBCDCVoltInf_V/1 -> OBCDCVoltInf/2
  [inp_CanValid_bus] -> slr1_10/1
  slr1_10/1 -> OBCDCVoltInf/3  "<VINP_CANMsgValidCCU1_flg>"
  OBCDCVoltInf/1 -> VINP_OBCDCVoltInf_V/1  "VINP_OBCDCVoltInf_V"
  OBCDCVoltInf/2 -> Terminator_10/1
  [BHAL_outputs] -> slr_VHAL_OBCPreCompleted_enum/1
  slr_VHAL_OBCPreCompleted_enum/1 -> OBCPreCompleted/1  "<VHAL_OBCPreCompleted_enum>"
  True_VHAL_OBCPreCompleted_enum/1 -> OBCPreCompleted/2
  [inp_CanValid_bus] -> slr1_11/1
  slr1_11/1 -> OBCPreCompleted/3  "<VINP_CANMsgValidCCU1_flg>"
  OBCPreCompleted/1 -> VINP_OBCPreCompleted_enum/1  "VINP_OBCPreCompleted_enum"
  OBCPreCompleted/2 -> Terminator_11/1
  [BHAL_outputs] -> slr_VHAL_OBCWakeup4Plugin_flg/1
  slr_VHAL_OBCWakeup4Plugin_flg/1 -> OBCWakeup4Plugin/1  "<VHAL_OBCWakeup4Plugin_flg>"
  True_VHAL_OBCWakeup4Plugin_flg/1 -> OBCWakeup4Plugin/2
  [inp_CanValid_bus] -> slr1_12/1
  slr1_12/1 -> OBCWakeup4Plugin/3  "<VINP_CANMsgValidCCU1_flg>"
  OBCWakeup4Plugin/1 -> VINP_OBCWakeup4Plugin_flg/1  "VINP_OBCWakeup4Plugin_flg"
  OBCWakeup4Plugin/2 -> Terminator_12/1
  [BHAL_outputs] -> slr_VHAL_RCCCU1_enum/1
  slr_VHAL_RCCCU1_enum/1 -> RCCCU1/1  "<VHAL_RCCCU1_enum>"
  True_VHAL_RCCCU1_enum/1 -> RCCCU1/2
  [inp_CanValid_bus] -> slr1_13/1
  slr1_13/1 -> RCCCU1/3  "<VINP_CANMsgValidCCU1_flg>"
  RCCCU1/1 -> VINP_RCCCU1_enum/1  "VINP_RCCCU1_enum"
  RCCCU1/2 -> Terminator_13/1
